simulink model "Model_Vehicle_Trailer"  (R2020a)
settings: Solver=FixedStepAuto  StartTime=0.0  StopTime=10.0  FixedStep=1e-3  RelTol=1e-3
undefined symbols (not defined in the file): l1, l12, l2, v
settings Model: Creator=uic26460  LastModifiedBy=uic26460

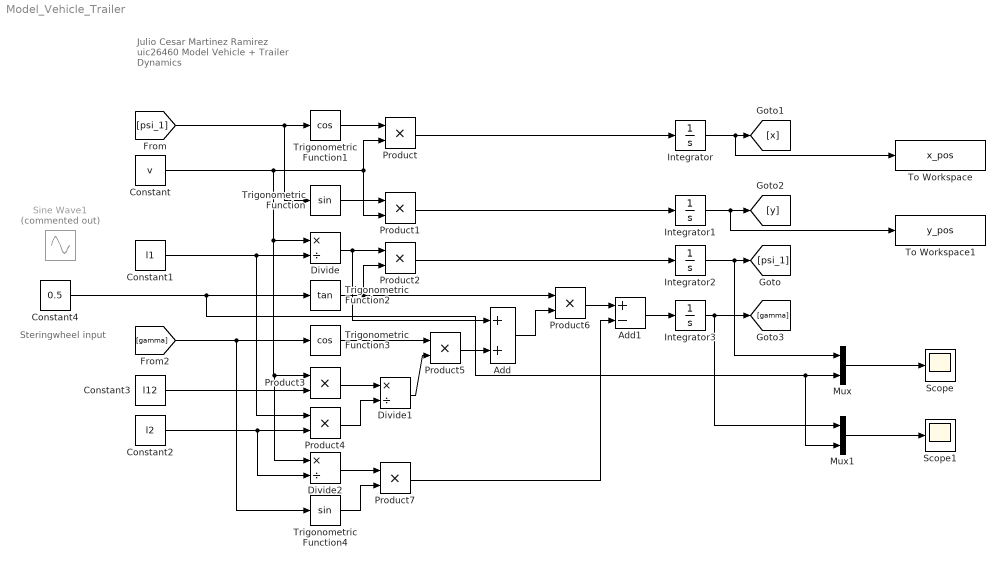
== system Model_Vehicle_Trailer ==
  note: Steringwheel input
  note: Julio Cesar Martinez Ramirez
      | uic26460
      | Model Vehicle + Trailer Dynamics
  Add : Sum
  Add1 : Sum  Inputs=+-
  Constant : Constant  Value=v
  Constant1 : Constant  Value=l1
  Constant2 : Constant  Value=l2
  Constant3 : Constant  Value=l12
  Constant4 : Constant  Value=0.5
  Divide : Product  Inputs=*/
  Divide1 : Product  Inputs=*/
  Divide2 : Product  Inputs=*/
  Integrator{,1..3} (4 alike) : Integrator
  Mux : Mux  Inputs=2
  Mux1 : Mux  Inputs=2
  Product{,1..7} (8 alike) : Product
  Scope : Scope
  Scope1 : Scope
  Sine Wave1 : Sin  Commented=on  Amplitude=0.2  Frequency=10  SampleTime=0
  To Workspace : ToWorkspace  VariableName=x_pos  SaveFormat=Timeseries  SampleTime=-1
  To Workspace1 : ToWorkspace  VariableName=y_pos  SaveFormat=Timeseries  SampleTime=-1
  Trigonometric Function : Trigonometry
  Trigonometric Function1 : Trigonometry  Operator=cos
  Trigonometric Function2 : Trigonometry  Operator=tan
  Trigonometric Function3 : Trigonometry  Operator=cos
  Trigonometric Function4 : Trigonometry
  wires:
  Trigonometric Function1/1 -> Product/1
  [psi_1] -> Trigonometric Function/1, Trigonometric Function1/1
  Constant/1 -> Divide2/1, Product3/1, Divide/1, Product1/2, Product/2
  Product/1 -> Integrator/1
  Product1/1 -> Integrator1/1
  Trigonometric Function/1 -> Product1/1
  Constant1/1 -> Product4/1, Divide/2
  Divide/1 -> Add/1, Product2/1
  Trigonometric Function2/1 -> Product2/2, Product6/1
  Constant4/1 -> Mux1/2, Mux/2, Trigonometric Function2/1
  Product2/1 -> Integrator2/1
  Integrator/1 -> To Workspace/1, [x]
  Integrator1/1 -> To Workspace1/1, [y]
  [gamma] -> Trigonometric Function4/1, Trigonometric Function3/1
  Constant3/1 -> Product3/2
  Constant2/1 -> Divide2/2, Product4/2
  Product3/1 -> Divide1/1
  Product4/1 -> Divide1/2
  Divide1/1 -> Product5/2
  Trigonometric Function3/1 -> Product5/1
  Product5/1 -> Add/2
  Add/1 -> Product6/2
  Product6/1 -> Add1/1
  Divide2/1 -> Product7/1
  Trigonometric Function4/1 -> Product7/2
  Product7/1 -> Add1/2
  Add1/1 -> Integrator3/1
  Integrator3/1 -> Mux1/1, [gamma]
  Integrator2/1 -> Mux/1, [psi_1]
  Mux/1 -> Scope/1
  Mux1/1 -> Scope1/1
